simulink model "quad_x_train"  (R2014b)
settings: Solver=ode45  StartTime=0.0  StopTime=10.0  RelTol=1e-3
libraries: neural x1
settings Model: Creator=ghost  LastModifiedBy=ghost

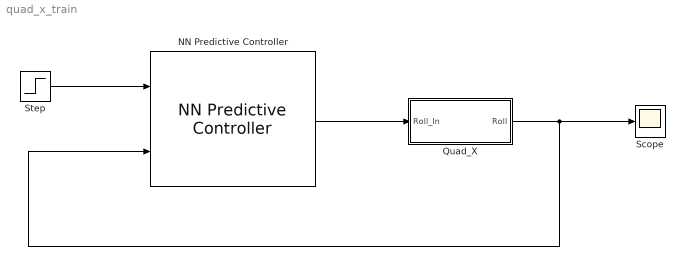
== system quad_x_train ==
  NN Predictive Controller : neural/Control Systems/NN Predictive Controller  epochs=800  minp=-0.99375627128259669  maxp=0.99718677655187538  mint=-11.476882979154116  maxt=0.99718677655187538  Normalize=1  IW=[0.039998660620629928 0.054319765832510608;-0.010503535501637755 -0.019695859789655188;-0.017929844429394222 -0.017987719633573145;-0.15873458599410625 -0.23890856720996989;-0.13484413942787421 -0.045556897178475317;0.55199711251037986 0.19357513454006872;-0.056128979769489128 -0.058493866282012606;-0.050041935554247574 -0.058676958961361075;-0.51342226469245844 -0.16103467717091358;0.094238526031955525 0.043982450778776931;-0.40690614066746572 -0.1378701762785233;-0.076058654609683224 -0.061051002773556594;-0.046552391771399686 -0.051023745907735764]  LW1_2=[-0.043314732256269188;-1.3295460339849443;-1.0162121533972843;0.0050899148605056252;-0.50042099070870627;-0.29434622763017254;0.035023037939621651;0.0388239235362587;0.0078823202382635755;-0.032637242251995033;-0.33184722281130602;0.017985074754463665;0.032846785601753907]  LW2_1=[-0.10107553326643129 -0.43152252561111648 -0.7651203191331083 -0.097639060643939693 -0.42820246096364367 -0.13049858893320174 0.1167072490731577 0.11487703456844785 -0.27200029396797054 -0.12790647778402289 0.26845125589846164 0.14095111255833445 0.09180920326466567]  B1=[-0.033707570801635167;-0.47549596614413381;0.94594550137361211;-0.044475986989229097;-0.0056021811866312742;0.20269094438666568;0.029333788248414833;0.034120233153385485;-0.10477809021971642;0.022819986520979749;-0.00087034047782172917;0.071614354293789095;0.02306375039488753]  B2=0.33893159470915019  max_i_int=0.1  min_i_int=0.005  limit_output=0  max_output=Inf  min_output=-Inf  Use_Previous_Weights=1  N2=4  Nu=3  Ts=0.01  rho=0.05  alpha=0.002  csrchfun=csrchbac  maxiter=2  S1=13  Ni=2  Nj=1  sim_file=quad_x_model  trainfun=trainbr  Use_validation=1  Use_Testing=1  max_i=1  min_i=-1  sam_training=800
  Quad_X : Subsystem  TreatAsAtomicUnit=on
  Scope : Scope
      settings: SaveName=ScopeData2
  Step : Step  SampleTime=0
  wires:
  Quad_X/1(Roll) -> NN Predictive Controller/2, Scope/1
  NN Predictive Controller/1 -> Quad_X/1(Roll_In)
  Step/1 -> NN Predictive Controller/1

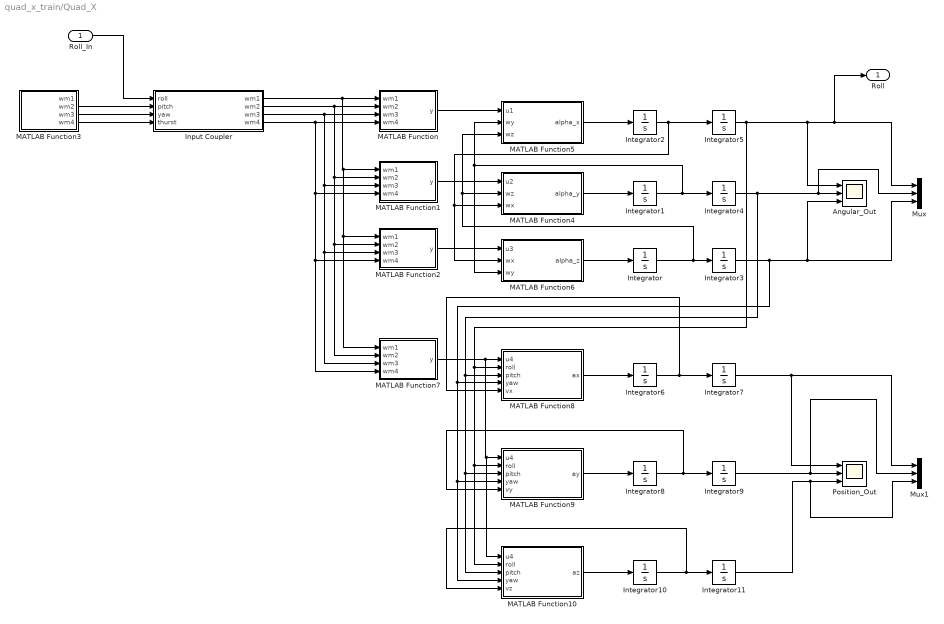
== system quad_x_train/Quad_X ==
  Roll_In : Inport
  Angular_Out : Scope  NumInputPorts=3
      settings: YMin=-5~-5~-5  YMax=5~5~5
  Input Coupler : MATLAB Function  TreatAsAtomicUnit=on
  Integrator{,1..11} (12 alike) : Integrator
  MATLAB Function : MATLAB Function  TreatAsAtomicUnit=on
  MATLAB Function1 : MATLAB Function  TreatAsAtomicUnit=on
  MATLAB Function10 : MATLAB Function  TreatAsAtomicUnit=on
  MATLAB Function2 : MATLAB Function  TreatAsAtomicUnit=on
  MATLAB Function3 : MATLAB Function  TreatAsAtomicUnit=on
  MATLAB Function4 : MATLAB Function  TreatAsAtomicUnit=on
  MATLAB Function5 : MATLAB Function  TreatAsAtomicUnit=on
  MATLAB Function6 : MATLAB Function  TreatAsAtomicUnit=on
  MATLAB Function7 : MATLAB Function  TreatAsAtomicUnit=on
  MATLAB Function8 : MATLAB Function  TreatAsAtomicUnit=on
  MATLAB Function9 : MATLAB Function  TreatAsAtomicUnit=on
  Mux : Mux  Inputs=3
  Mux1 : Mux  Inputs=3
  "Position_Out " : Scope  NumInputPorts=3
      settings: YMin=-5~-5~-5  YMax=5~5~5
  Roll : Outport
  wires:
  Input Coupler/1(wm1) -> MATLAB Function7/1(wm1), MATLAB Function2/1(wm1), MATLAB Function1/1(wm1), MATLAB Function/1(wm1)
  Input Coupler/2(wm2) -> MATLAB Function7/2(wm2), MATLAB Function2/2(wm2), MATLAB Function1/2(wm2), MATLAB Function/2(wm2)
  Input Coupler/3(wm3) -> MATLAB Function7/3(wm3), MATLAB Function2/3(wm3), MATLAB Function1/3(wm3), MATLAB Function/3(wm3)
  Input Coupler/4(wm4) -> MATLAB Function7/4(wm4), MATLAB Function2/4(wm4), MATLAB Function1/4(wm4), MATLAB Function/4(wm4)
  MATLAB Function1/1(y) -> MATLAB Function4/1(u2)
  MATLAB Function2/1(y) -> MATLAB Function6/1(u3)
  MATLAB Function6/1(alpha_z) -> Integrator/1
  Integrator/1 -> Integrator3/1, MATLAB Function5/3(wz), MATLAB Function4/2(wz)
  MATLAB Function5/1(alpha_x) -> Integrator2/1
  MATLAB Function4/1(alpha_y) -> Integrator1/1
  Integrator2/1 -> MATLAB Function6/2(wx), MATLAB Function4/3(wx), Integrator5/1
  Integrator1/1 -> MATLAB Function5/2(wy), MATLAB Function6/3(wy), Integrator4/1
  Integrator3/1 -> MATLAB Function10/4(yaw), MATLAB Function9/4(yaw), MATLAB Function8/4(yaw), Angular_Out/3, Mux/3
  Integrator4/1 -> Mux/2, Angular_Out/2, MATLAB Function10/3(pitch), MATLAB Function9/3(pitch), MATLAB Function8/3(pitch)
  MATLAB Function/1(y) -> MATLAB Function5/1(u1)
  MATLAB Function8/1(ax) -> Integrator6/1
  Integrator6/1 -> MATLAB Function8/5(vx), Integrator7/1
  MATLAB Function7/1(y) -> MATLAB Function10/1(u4), MATLAB Function9/1(u4), MATLAB Function8/1(u4)
  MATLAB Function9/1(ay) -> Integrator8/1
  Integrator8/1 -> MATLAB Function9/5(vy), Integrator9/1
  MATLAB Function10/1(az) -> Integrator10/1
  Integrator10/1 -> MATLAB Function10/5(vz), Integrator11/1
  Integrator5/1 -> MATLAB Function10/2(roll), MATLAB Function9/2(roll), MATLAB Function8/2(roll), Angular_Out/1, Roll/1, Mux/1
  Integrator7/1 -> "Position_Out "/1, Mux1/1
  Integrator9/1 -> Mux1/2, "Position_Out "/2
  Integrator11/1 -> Mux1/3, "Position_Out "/3
  Roll_In/1 -> Input Coupler/1(roll)
  MATLAB Function3/2(wm2) -> Input Coupler/2(pitch)
  MATLAB Function3/3(wm3) -> Input Coupler/3(yaw)
  MATLAB Function3/4(wm4) -> Input Coupler/4(thurst)

== matlab function quad_x_train/Quad_X/MATLAB Function1 ==
  data: wm1 input; y output; wm2 input; wm3 input; wm4 input
function y = u2(wm1, wm2, wm3, wm4)
%#codegen

k1 = 3.1 * 10^-7;
y = k1 * (wm2^2 + wm4^2 - wm1^2 - wm3^2);
return;

== matlab function quad_x_train/Quad_X/MATLAB Function ==
  data: wm1 input; y output; wm2 input; wm3 input; wm4 input
function y = u1(wm1, wm2, wm3, wm4)
%#codegen

k1 = 3.1 * 10^-7;
y = k1 * (wm2^2 + wm3^2 - wm1^2 - wm4^2);
return;

== matlab function quad_x_train/Quad_X/MATLAB Function2 ==
  data: wm1 input; y output; wm2 input; wm3 input; wm4 input
function y = u3(wm1, wm2, wm3, wm4)
%#codegen

k2 = 3.1 * 10^-7;
y = k2 * (wm1^2 + wm2^2 - wm3^2 - wm4^2);
return;

== matlab function quad_x_train/Quad_X/Input Coupler ==
  data: roll input; wm1 output; pitch input; yaw input; thurst input; wm2 output; wm3 output; wm4 output
function [wm1, wm2, wm3, wm4] = input_coupler(roll, pitch, yaw, thurst)
%#codegen

% 控制耦合
% 输入是归一化的，-1~1

% 基础输入 1000
thurst_bias = 1407;

% 去归一化
roll  = roll  * 500;
pitch = pitch * 500;
yaw   = yaw   * 500;
thurst = thurst * 1000;

wm1 = thurst + thurst_bias - roll - pitch + yaw;
wm2 = thurst + thurst_bias + roll + pitch + yaw;
wm3 = thurst + thurst_bias + roll - pitch - yaw;
wm4 = thurst + thurst_bias - roll + pitch - yaw;


return;

== matlab function quad_x_train/Quad_X/MATLAB Function4 ==
  data: u2 input; wz input; alpha_y output; wx input
function alpha_y = calc_pitch_a(u2, wz, wx)
%#codegen

l = 0.25;
Jx = 0.033;
Jy = 0.033;
Jz = 0.061;

alpha_y = u2 * (sqrt(2) / 2) * l + (Jz - Jx) * wz * wx;
alpha_y = alpha_y / Jy;


return;

== matlab function quad_x_train/Quad_X/MATLAB Function5 ==
  data: u1 input; wy input; wz input; alpha_x output
function alpha_x = calc_roll_a(u1, wy, wz)
%#codegen

l = 0.25;
Jx = 0.033;
Jy = 0.033;
Jz = 0.061;

alpha_x = u1 * (sqrt(2) / 2) * l + (Jy - Jz) * wy * wz;
alpha_x = alpha_x / Jx;


return;

== matlab function quad_x_train/Quad_X/MATLAB Function6 ==
  data: u3 input; wx input; alpha_z output; wy input
function alpha_z = calc_yaw_a(u3, wx, wy)
%#codegen

l = 0.25;
Jx = 0.033;
Jy = 0.033;
Jz = 0.061;

alpha_z = u3 * l + (Jx - Jy) * wx * wy;
alpha_z = alpha_z / Jz;


return;

== matlab function quad_x_train/Quad_X/MATLAB Function7 ==
  data: wm1 input; y output; wm2 input; wm3 input; wm4 input
function y = u4(wm1, wm2, wm3, wm4)
%#codegen

k1 = 3.1 * 10^-7;
y = k1 * (wm1^2 + wm2^2 + wm3^2 + wm4^2);
return;

== matlab function quad_x_train/Quad_X/MATLAB Function8 ==
  data: u4 input; roll input; pitch input; ax output; yaw input; vx input
function ax = calc_ax(u4, roll, pitch, yaw, vx)
%#codegen
% roll  -> alpha
% pitch -> beta
% yaw   -> gamma

m  = 0.25;
g  = 9.81;
kf = 0;

ax = u4 * (sin(roll) * sin(yaw) + cos(roll) * sin(pitch) * cos(yaw));
ax = ax - kf * vx;
ax = ax / m;

return;

== matlab function quad_x_train/Quad_X/MATLAB Function9 ==
  data: u4 input; roll input; pitch input; ay output; yaw input; vy input
function ay = calc_ay(u4, roll, pitch, yaw, vy)
%#codegen
% roll  -> alpha
% pitch -> beta
% yaw   -> gamma

m  = 0.25;
g  = 9.81;
kf = 0;

ay = u4 * (-sin(roll) * cos(yaw) + cos(roll) * sin(pitch) * sin(yaw));
ay = ay - kf * vy;
ay = ay / m;

return;

== matlab function quad_x_train/Quad_X/MATLAB Function10 ==
  data: u4 input; roll input; pitch input; az output; yaw input; vz input
function az = calc_az(u4, roll, pitch, yaw, vz)
%#codegen
% roll  -> alpha
% pitch -> beta
% yaw   -> gamma

m  = 0.25;
g  = 9.81;
kf = 0;

az = u4 * (cos(roll) * cos(pitch));
az = az / m - g;

return;

== matlab function quad_x_train/Quad_X/MATLAB Function3 ==
  data: wm1 output; wm2 output; wm3 output; wm4 output
function [wm1, wm2, wm3, wm4] = fcn
%#codegen

% 1406 - 1407平飞

wm1 = 0;
wm2 = 0;
wm3 = 0;
wm4 = 0;
